simulink model "untitled"  (R2012b)
settings: Solver=ode45  StartTime=0.0  StopTime=10  RelTol=1e-3
values from neighbouring files (symbols this model uses):
  A = [1.2 -3.7 ; 2.2 -1.5]    [config.m]
  B = [0.33 1.1 ; -2 0.5]    [config.m]
  C = [1 0]    [config.m]
  L = L'    [config.m]
  Ts = 0.03    [config.m]
undefined symbols (not defined in the file): sysd
libraries: simulink x1
settings Model: Creator=Juliano  LastModifiedBy=Juliano
settings OptimizationCC: InlineParams=on

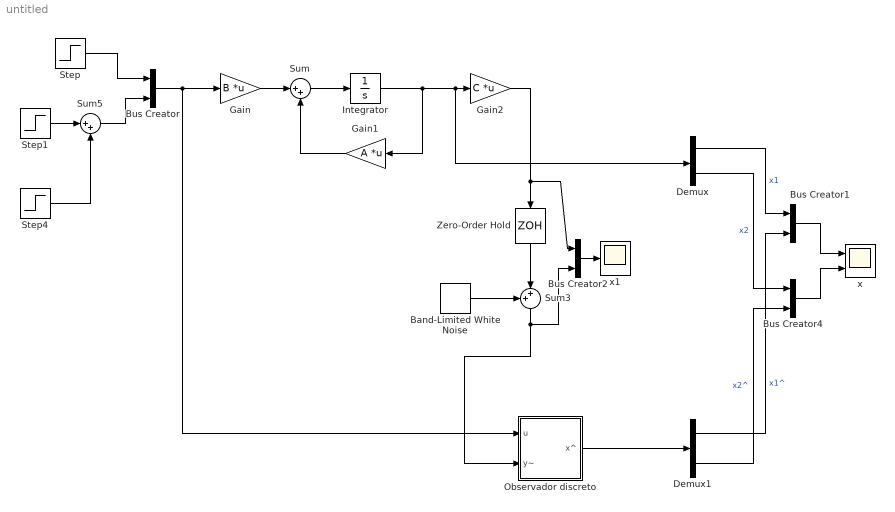
== system untitled ==
  Band-Limited White Noise : simulink/Sources/Band-Limited White Noise  Cov=[0.0005]  Ts=Ts  seed=[23341]
  Bus Creator{,1..2,4} (4 alike) : BusCreator  Inputs=2
  Demux : Demux  Outputs=2
  Demux1 : Demux  Outputs=2
  Gain : Gain  Gain=B  Multiplication=Matrix(K*u)
  Gain1 : Gain  Gain=A  Multiplication=Matrix(K*u)
  Gain2 : Gain  Gain=C  Multiplication=Matrix(K*u)
  Integrator : Integrator
  Observador discreto : Subsystem  mask{Ahat=sysd.a, Bhat=sysd.b, C=sysd.c, L=L}
      mask prompts: Ahat "Estimativa de A"; Bhat "Estimativa de B"
  Step : Step  Time=0  SampleTime=0
  Step1 : Step  After=10  SampleTime=0
  Step4 : Step  Time=4  After=-20  SampleTime=0
  Sum : Sum  Inputs=|++
  Sum3 : Sum  Inputs=++|
  Sum5 : Sum  Inputs=|++
  Zero-Order Hold : ZeroOrderHold  SampleTime=Ts
  x : Scope  NumInputPorts=2
      settings: ShowLegends=on  YMin=-5~-5  YMax=5~5  SaveName=ScopeData2
  x1 : Scope
      settings: ShowLegends=on
  wires:
  Step/1 -> Bus Creator/1
  Gain/1 -> Sum/1
  Sum/1 -> Integrator/1
  Gain1/1 -> Sum/2
  Integrator/1 -> Demux/1, Gain2/1, Gain1/1
  Bus Creator1/1 -> x/1
  Bus Creator4/1 -> x/2
  Demux/1 -> Bus Creator1/1  "x1"
  Demux1/1 -> Bus Creator1/2  "x1^"
  Demux/2 -> Bus Creator4/1  "x2"
  Demux1/2 -> Bus Creator4/2  "x2^"
  Step1/1 -> Sum5/1
  Sum5/1 -> Bus Creator/2
  Step4/1 -> Sum5/2
  Sum3/1 -> Observador discreto/2(y~), Bus Creator2/2
  Gain2/1 -> Bus Creator2/1, Zero-Order Hold/1
  Zero-Order Hold/1 -> Sum3/2
  Bus Creator2/1 -> x1/1
  Observador discreto/1(x^) -> Demux1/1
  Bus Creator/1 -> Observador discreto/1(u), Gain/1
  Band-Limited White Noise/1 -> Sum3/1

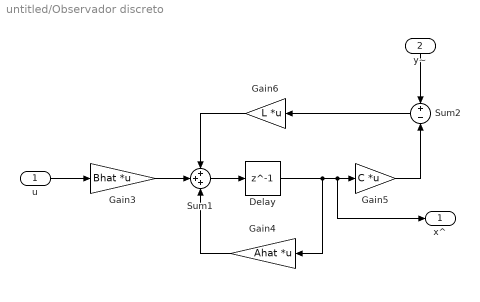
== system untitled/Observador discreto ==
  u : Inport
  y~ : Inport  Port=2
  Delay : Delay  DelayLength=1  SampleTime=Ts
  Gain3 : Gain  Gain=Bhat  Multiplication=Matrix(K*u)
  Gain4 : Gain  Gain=Ahat  Multiplication=Matrix(K*u)
  Gain5 : Gain  Gain=C  Multiplication=Matrix(K*u)
  Gain6 : Gain  Gain=L  Multiplication=Matrix(K*u)
  Sum1 : Sum  Inputs=+++
  Sum2 : Sum  Inputs=+-
  x^ : Outport
  wires:
  Gain3/1 -> Sum1/2
  Gain4/1 -> Sum1/3
  Gain6/1 -> Sum1/1
  Sum2/1 -> Gain6/1
  Delay/1 -> Gain4/1, x^/1, Gain5/1
  Gain5/1 -> Sum2/2
  Sum1/1 -> Delay/1
  y~/1 -> Sum2/1
  u/1 -> Gain3/1
